simulink model "messaging"  (R2023b)
settings: Solver=FixedStepAuto  StartTime=0.0  StopTime=12.5  FixedStep=.1  RelTol=1e-3
settings Model: Creator=Yasmine Adler  LastModifiedBy=Yasmine Adler

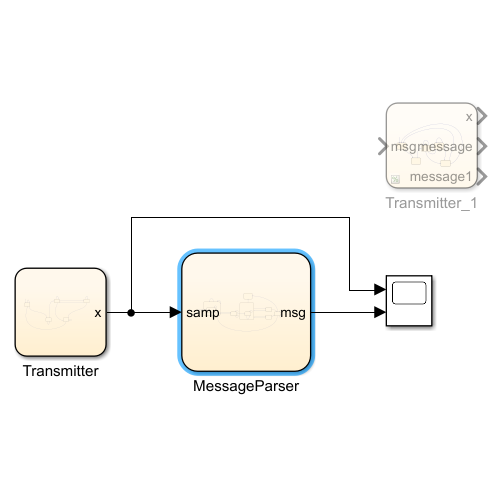
[thumbnail: Simulink's stored preview of the top-level diagram]
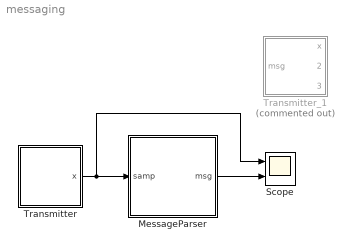
== system messaging ==
  MessageParser : Stateflow chart  TreatAsAtomicUnit=on
  Scope : Scope  NumInputPorts=2
  Transmitter : Stateflow chart  TreatAsAtomicUnit=on
  Transmitter_1 : Stateflow chart  Commented=on  TreatAsAtomicUnit=on
  wires:
  MessageParser/1(msg) -> Scope/2
  Transmitter/1(x) -> Scope/1, MessageParser/1(samp)

== stateflow chart messaging/MessageParser ==
  state errorState
    msg=3
  state SYNCH
    state synchronize
      state synchronizeSample
      synchronizeSample -> synchronizeSample [order 1] : [samp==1]{ctr = ctr + 1, onectr = onectr + 1}
      synchronizeSample -> synchronizeSample [order 2] : [samp==0]{ctr = ctr + 1}
    state startSample
    synchronize -> synchronize [order 3] : [ctr==3&&onectr<3&&samp==0]{ctr=0, onectr=0, zeroctr=0}
    synchronize -> synchronize [order 2] : [onectr>=3&&ctr==4&&samp==1]{bitctr = bitctr + 1;onectr=0;zeroctr=0;ctr=0}
    startSample -> startSample [order 1] : [samp==0]{zeroctr = zeroctr + 1, ctr = ctr + 1}
    synchronize -> startSample [order 1] : [bitctr == preambleLen]{ctr=0, onectr=0}
    startSample -> synchronize [order 4] : [zeroctr>=4&&ctr==5]{zeroctr=0,ctr=0}
    startSample -> startSample [order 3] : [samp==1]{ctr = ctr + 1}
  state MESSAGE
    state msgbytes
      state msgSample
      msgSample -> msgSample [order 1] : [samp==0]{zeroctr = zeroctr + 1, ctr = ctr + 1}
      msgSample -> msgSample [order 2] : [samp==1]{ctr = ctr + 1,onectr = onectr + 1}
    state printOne
      msg=1
    state printZero1
      msg=0
    msgbytes -> printOne [order 2] : [ctr==4&&(onectr+samp>=4)]{bitctr = bitctr + 1}
    printOne -> msgbytes [order 2] : {onectr=0;zeroctr=0;ctr=0;msg=3}
    msgbytes -> printZero1 [order 1] : [ctr==4&&(onectr+samp)<=1]{bitctr = bitctr + 1}
    printZero1 -> msgbytes [order 2] : {onectr=0;zeroctr=0;ctr=0;msg=3}
  state CRC
    state crcSample
    crcSample -> crcSample [order 2] : [samp==0]{ctr = ctr + 1;zeroctr = zeroctr + 1}
    crcSample -> crcSample [order 3] : [samp==1]{ctr = ctr + 1}
  crcSample -> errorState [order 1] : [ctr==5&&zeroctr<4]
  msgbytes -> errorState [order 3] : [ctr==4]
  printOne -> crcSample [order 1] : [bitctr==8]{onectr=0;zeroctr=0;ctr=0;bitctr=0;msg=3}
  printZero1 -> crcSample [order 1] : [bitctr==8]{onectr=0;zeroctr=0;ctr=0;bitctr=0;msg=3}
  (default) -> synchronizeSample : {onectr=0;msg=3;ctr=0;bitctr=0;zeroctr=0;bit=0}
  crcSample -> synchronize [order 4] : [ctr==5&&zeroctr>=4]{zeroctr=0; ctr=0}
  startSample -> msgSample [order 2] : [zeroctr>=4&&ctr==5]{zeroctr=0,ctr=0;bitctr=0}
  data: samp input; onectr local; ctr local; preambleLen constant double =8; bitctr local; msg output; bit local; zeroctr local

== stateflow chart messaging/Transmitter_1 ==
  state preamble
    x = 11111111
  state bitstream0
    x = 0
  state bitstream
    x = msg(y)
  state start
    x = 0
  state crc
    x = 0
  note: TODO: build the CRC function in Matlab and link
  crc -> preamble [order 1] : [y >= strlength(msg)]{y=0}
  crc -> preamble [order 2] : [y<strlength(msg)]
  (default) -> preamble : {y=0}
  bitstream0 -> bitstream0 [order 2] : [mod(y,packlen)~=0]{y = y + 1}
  bitstream -> bitstream [order 3] : [mod(y,packlen)~=0 && y< strlength(msg)]{y = y + 1}
  bitstream0 -> crc [order 1] : [mod(y,packlen)==0]
  start -> bitstream
  preamble -> start
  bitstream -> bitstream0 [order 2] : [(mod(y,packlen)~=0)&&(y>= strlength(msg))]{y = y + 1}
  bitstream -> crc [order 1] : [mod(y,packlen) == 0]
  data: msg input; x output; y local; packlen constant double =8; message output; message1 output

== stateflow chart messaging/Transmitter ==
  state bitstream1
    x = 1
  state bitstream0
    x = 0
  state preamble
    x = 1
  state start
    x = 0
  state crc
    x = 0
  bitstream0 -> bitstream0 [order 3] : {sampCount = sampCount + 1}
  bitstream1 -> bitstream1 [order 3] : {sampCount = sampCount + 1}
  (default) -> preamble : {x=0; bitcount = 0; sampCount = 0}
  preamble -> preamble [order 2] : [sampCount<preambleLen*samp_per_bit]{sampCount = sampCount + 1}
  bitstream1 -> bitstream0 [order 2] : [sampCount==samp_per_bit]{sampCount=0; bitcount = bitcount + 1}
  start -> bitstream1 [order 1] : [sampCount==samp_per_bit]{bitcount=0, sampCount=0}
  bitstream0 -> bitstream1 [order 2] : [sampCount==samp_per_bit]{sampCount=0; bitcount = bitcount + 1}
  bitstream1 -> crc [order 1] : [bitcount==msgLen-1]
  bitstream0 -> crc [order 1] : [bitcount==msgLen-1]{sampCount=0}
  crc -> preamble [order 1] : [sampCount==samp_per_bit]{bitcount=0; sampCount=0}
  preamble -> start [order 1] : [sampCount==preambleLen*samp_per_bit]{sampCount=0}
  crc -> crc [order 2] : [sampCount<samp_per_bit]{sampCount = sampCount + 1}
  start -> start [order 2] : {sampCount = sampCount + 1}
  data: x output; preambleLen constant double =8; bitcount local; samp_per_bit constant double =5; msgLen constant double =8; sampCount local
